simulink model "WeightOnWheelLatch"  (R2021b)
settings: Solver=FixedStepDiscrete  StartTime=0.0  StopTime=10.0  FixedStep=1/10  RelTol=1e-3
settings Model: Creator=david  LastModifiedBy=david

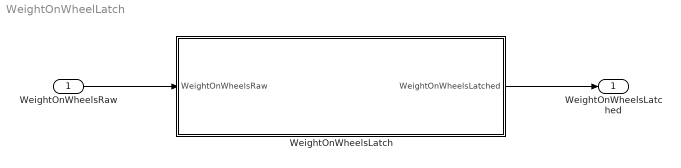
== system WeightOnWheelLatch ==
  WeightOnWheelsRaw : Inport  OutDataTypeStr=boolean
  WeightOnWheelsLatch : Stateflow chart  TreatAsAtomicUnit=on
  WeightOnWheelsLatched : Outport  OutDataTypeStr=boolean
  wires:
  WeightOnWheelsRaw/1 -> WeightOnWheelsLatch/1(WeightOnWheelsRaw)
  WeightOnWheelsLatch/1(WeightOnWheelsLatched) -> WeightOnWheelsLatched/1

== stateflow chart WeightOnWheelLatch/WeightOnWheelsLatch ==
  state WeightOnWheelsEntry
    WeightOnWheelsLatched = false;
  state LatchRejected
    entry:
    WeightOnWheelsLatched = false;
  state SignalLatched
    entry:
    WeightOnWheelsLatched = true;
  (default) -> WeightOnWheelsEntry
  SignalLatched -> WeightOnWheelsEntry : [WeightOnWheelsRaw == false]
  WeightOnWheelsEntry -> (junction 10) [order 1] : [WeightOnWheelsRaw == true]
  LatchRejected -> WeightOnWheelsEntry : [WeightOnWheelsRaw == true]
  WeightOnWheelsEntry -> LatchRejected [order 2] : [WeightOnWheelsRaw == false]
  (junction 10) -> SignalLatched : [after(3, sec)]
  data: WeightOnWheelsLatched output; WeightOnWheelsRaw input
